simulink model "circularROE_J2"  (R2023a)
settings: Solver=ode4  StartTime=0.0  StopTime=10.0  FixedStep=dt  RelTol=1e-3
settings Model: Creator=ndelurgio  LastModifiedBy=ndelurgio

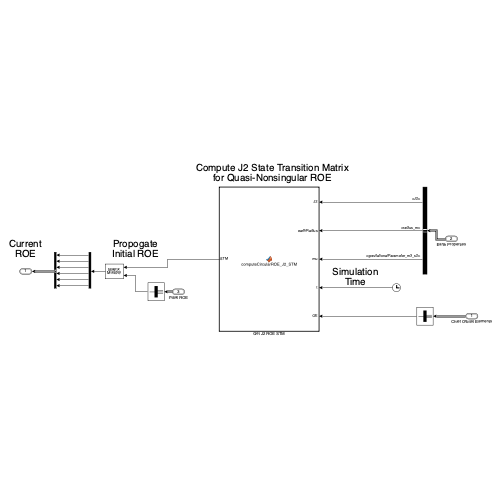
[thumbnail: Simulink's stored preview of the top-level diagram]
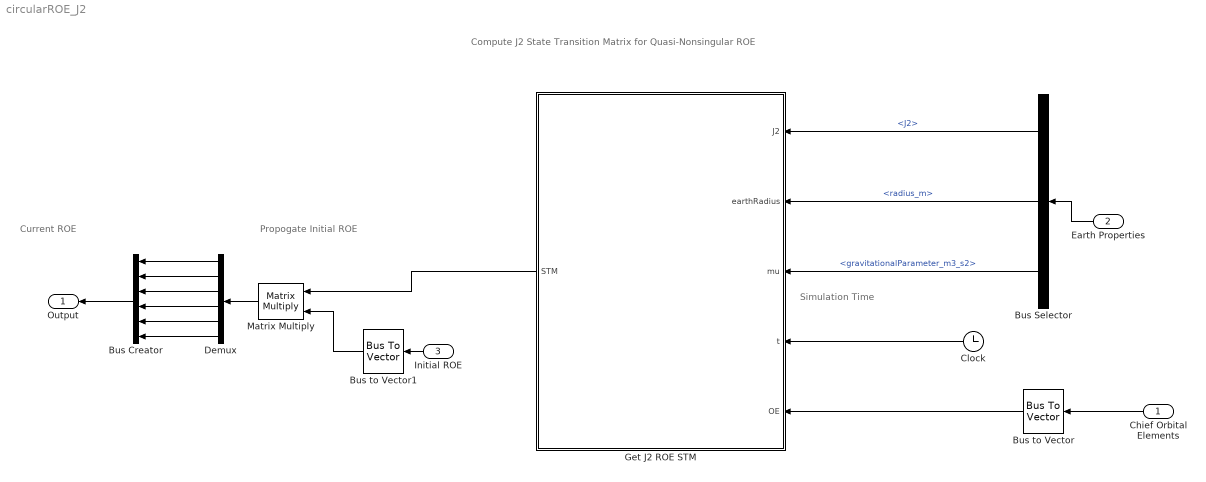
== system circularROE_J2 ==
  note: Compute J2 State Transition Matrix for Quasi-Nonsingular ROE
  note: Propogate Initial ROE
  note: Simulation Time
  note: Current ROE
  Chief Orbital Elements : Inport  OutDataTypeStr=Bus: meanOrbitElements
  Earth Properties : Inport  Port=2  OutDataTypeStr=Bus: earthProperties
  Initial ROE : Inport  Port=3  OutDataTypeStr=Bus: damicoROE
  Bus Creator : BusCreator  Inputs=6  OutDataTypeStr=Bus: damicoROE
  Bus Selector : BusSelector  OutputSignals=J2,radius_m,gravitationalParameter_m3_s2
  Bus to Vector : BusToVector
  Bus to Vector1 : BusToVector
  Clock : Clock
  Demux : Demux  Outputs=6
  Get J2 ROE STM : MATLAB Function  TreatAsAtomicUnit=on
  Matrix Multiply : Product  Multiplication=Matrix(*)
  Output : Outport  OutDataTypeStr=Bus: damicoROE
  wires:
  Chief Orbital Elements/1 -> Bus to Vector/1
  Bus to Vector/1 -> Get J2 ROE STM/5(OE)
  Earth Properties/1 -> Bus Selector/1
  Bus Selector/1 -> Get J2 ROE STM/1(J2)  "<J2>"
  Bus Selector/2 -> Get J2 ROE STM/2(earthRadius)  "<radius_m>"
  Bus Selector/3 -> Get J2 ROE STM/3(mu)  "<gravitationalParameter_m3_s2>"
  Clock/1 -> Get J2 ROE STM/4(t)
  Get J2 ROE STM/1(STM) -> Matrix Multiply/1
  Demux/4 -> Bus Creator/4
  Demux/1 -> Bus Creator/1
  Demux/3 -> Bus Creator/3
  Demux/5 -> Bus Creator/5
  Demux/6 -> Bus Creator/6
  Demux/2 -> Bus Creator/2
  Bus Creator/1 -> Output/1
  Matrix Multiply/1 -> Demux/1
  Initial ROE/1 -> Bus to Vector1/1
  Bus to Vector1/1 -> Matrix Multiply/2

== matlab function circularROE_J2/Get J2 ROE STM ==
  data: J2 input; earthRadius input; mu input; t input; OE input; STM output
function STM = computeCircularROE_J2_STM(J2,earthRadius,mu,t,OE)
STM = computeCircularROE_J2_STM(OE,J2,earthRadius,mu,t);
end
